simulink model "lyap1"  (R2015a)
settings: Solver=ode45  StartTime=0.0  StopTime=10.0  RelTol=1e-3
values from neighbouring files (symbols this model uses):
  A = [0 -5 ... (first row only)    [test1.m]    (also in test2.m)
  P = lyap(A',Q)    [test1.m]    (also in test2.m)
  x0 = [1 0]'    [test2.m]
settings Model: Creator=shohei  LastModifiedBy=shohei

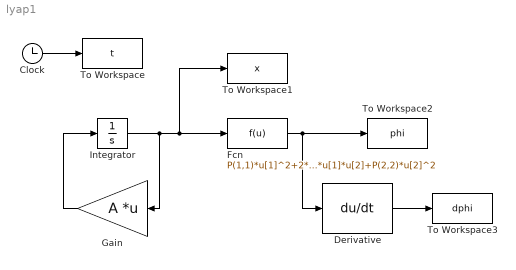
== system lyap1 ==
  Clock : Clock
  Derivative : Derivative
  Fcn : Fcn  Expr=P(1,1)*u[1]^2+2*P(1,2)*u[1]*u[2]+P(2,2)*u[2]^2
  Gain : Gain  Gain=A  Multiplication=Matrix(K*u)
  Integrator : Integrator  InitialCondition=x0
  To Workspace : ToWorkspace  VariableName=t  SampleTime=-1
  To Workspace1 : ToWorkspace  VariableName=x  SampleTime=-1
  To Workspace2 : ToWorkspace  VariableName=phi  SampleTime=-1
  To Workspace3 : ToWorkspace  VariableName=dphi  SampleTime=-1
  wires:
  Clock/1 -> To Workspace/1
  Gain/1 -> Integrator/1
  Integrator/1 -> Gain/1, To Workspace1/1, Fcn/1
  Fcn/1 -> Derivative/1, To Workspace2/1
  Derivative/1 -> To Workspace3/1
